simulink model "tp395815"  (Simulink 3.0)
settings: Solver=ode1  SolverMode=SingleTasking  StartTime=0.0  StopTime=inf  FixedStep=1  RelTol=1e-3  AbsTol=1e-6
libraries: udaq28LT_lib x1
settings Model: Creator=dmedonza  LastModifiedBy=mato  SaveFormat=Matrix  RTWTemplateMakefile=grt_vc.tmf  RTWOptions="-aEnforceIntegerDowncast=1 -aExtMode=0 -aExtModeTesting=0 -aFoldNonRolledExpr=1 -aForceParamTrailComments=0 -aGenerateComments=1 -aGenerateReport=0 -aIgnoreCustomStorageClasses=1 -aIncDataTypeInIds=0 -aIncHierarchyInIds=0 -aInlineInvariantSignals=0 -aInlinedPrmAccess=\"Literals\" -aLocalBlockOutputs=1 -aLogVarNameModifier=\"rt_\" -aMaxRTWIdLen=31 -aPrefixModelToSubsysFcnNames=1 -aRTWVerbose=1 -aRollThreshold=5 -aShowEliminatedStatements=0"

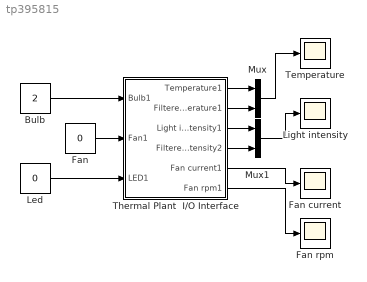
== system tp395815 ==
  Bulb : Constant  Value=2
  Fan : Constant  Value=0
  Fan current : Scope
      settings: TickLabels=on  TimeRange=auto  YMin=26  YMax=40  SaveName=y5  DataFormat=Matrix
  Fan rpm : Scope
      settings: TickLabels=on  TimeRange=100  YMin=0  YMax=6100  SaveName=y6  DataFormat=Matrix
  Led : Constant  Value=0
  Light intensity : Scope
      settings: TickLabels=on  TimeRange=100  YMin=0  YMax=90  SaveName=y34  DataFormat=Matrix
  Mux : Mux  Inputs=2
  Mux1 : Mux  Inputs=2
  Temperature : Scope
      settings: TickLabels=on  TimeRange=100  YMin=18  YMax=45  SaveName=y12  DataFormat=Matrix
  Thermal Plant  I/O Interface : Subsystem
      mask Display: disp('Thermo-optical\nPlant\nI/O Interface')
  wires:
  Mux/1 -> Temperature/1
  Mux1/1 -> Light intensity/1
  Bulb/1 -> Thermal Plant  I/O Interface/1(Bulb1)
  Fan/1 -> Thermal Plant  I/O Interface/2(Fan1)
  Led/1 -> Thermal Plant  I/O Interface/3(LED1)
  Thermal Plant  I/O Interface/1(Temperature1) -> Mux/1
  Thermal Plant  I/O Interface/2(Filtered  temperature1) -> Mux/2
  Thermal Plant  I/O Interface/3(Light intensity1) -> Mux1/1
  Thermal Plant  I/O Interface/4(Filtered  light intensity2) -> Mux1/2
  Thermal Plant  I/O Interface/5(Fan current1) -> Fan current/1
  Thermal Plant  I/O Interface/6(Fan rpm1) -> Fan rpm/1

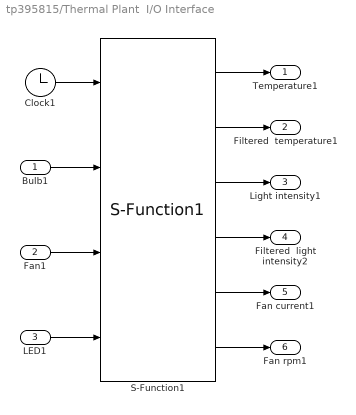
== system tp395815/Thermal Plant  I/O Interface ==
  Bulb1 : Inport  Port=1  PortWidth=-1  SampleTime=-1  DataType=auto
      settings: SignalType=auto
  Fan1 : Inport  Port=2  PortWidth=-1  SampleTime=-1  DataType=auto
      settings: SignalType=auto
  LED1 : Inport  Port=3  PortWidth=-1  SampleTime=-1  DataType=auto
      settings: SignalType=auto
  Clock1 : Clock
      settings: DisplayTime=off  Decimation=10
  S-Function1 : udaq28LT_lib/S-Function1  Priority=1  com_port=COM3  Ts=1  events_ot=5  rd_timeout=80  matlab_prior=HIGH_PRIORITY  warning=on  printout=off
  Temperature1 : Outport  Port=1
  Filtered  temperature1 : Outport  Port=2
  Light intensity1 : Outport  Port=3
  Filtered  light intensity2 : Outport  Port=4
  Fan current1 : Outport  Port=5
  Fan rpm1 : Outport  Port=6
  wires:
  S-Function1/1 -> Temperature1/1
  S-Function1/2 -> Filtered  temperature1/1
  Clock1/1 -> S-Function1/1
  Bulb1/1 -> S-Function1/2
  Fan1/1 -> S-Function1/3
  S-Function1/3 -> Light intensity1/1
  S-Function1/4 -> Filtered  light intensity2/1
  S-Function1/5 -> Fan current1/1
  S-Function1/6 -> Fan rpm1/1
  LED1/1 -> S-Function1/4
